simulink model "robot"  (R2018a)
settings: Solver=VariableStepAuto  StartTime=0.0  StopTime=5  RelTol=1e-3
values from neighbouring files (symbols this model uses):
  Ko = 1    [data_robot.m]
  Kv = 1    [data_robot.m]
  L = 0.02    [data_maglev.m]    (also in data_robot.m = 15)
  x0 = 10    [data_robot.m]
  y0 = 30    [data_robot.m]    (also in quadcopter optimisation.m = [0, 0]'; t1.m = 0)
settings Model: Creator=st006736  LastModifiedBy=Anton

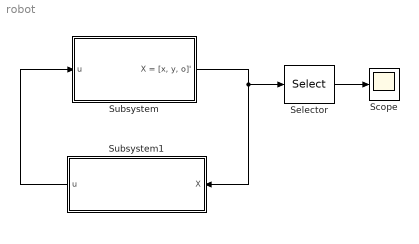
== system robot ==
  Scope : Scope
  Selector : Selector  InputPortWidth=3  IndexOptions=Index vector (dialog)  Indices=[1 2]  OutputSizes=1
  Subsystem : Subsystem
  Subsystem1 : Subsystem
  wires:
  Subsystem/1("X = [x, y, o]'") -> Selector/1, Subsystem1/1(X)
  Subsystem1/1(u) -> Subsystem/1(u)
  Selector/1 -> Scope/1

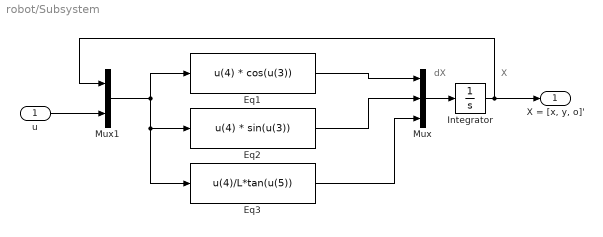
== system robot/Subsystem ==
  note: dX
  note: X
  u : Inport
  Eq1 : Fcn  Expr=u(4) * cos(u(3))
  Eq2 : Fcn  Expr=u(4) * sin(u(3))
  Eq3 : Fcn  Expr=u(4)/L*tan(u(5))
  Integrator : Integrator
  Mux : Mux  Inputs=3
  Mux1 : Mux  Inputs=2
  "X = [x, y, o]'" : Outport
  wires:
  Integrator/1 -> "X = [x, y, o]'"/1, Mux1/1
  Mux/1 -> Integrator/1
  Eq1/1 -> Mux/1
  Eq2/1 -> Mux/2
  Eq3/1 -> Mux/3
  u/1 -> Mux1/2
  Mux1/1 -> Eq1/1, Eq3/1, Eq2/1

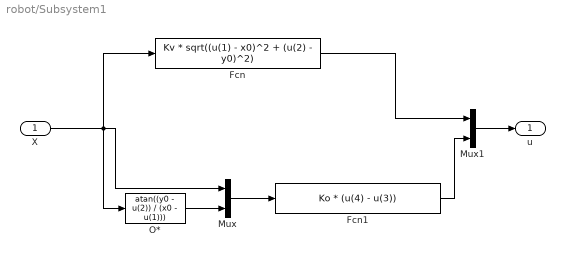
== system robot/Subsystem1 ==
  X : Inport
  Fcn : Fcn  Expr=Kv * sqrt((u(1) - x0)^2 + (u(2) - y0)^2)
  Fcn1 : Fcn  Expr=Ko * (u(4) - u(3))
  Mux : Mux  Inputs=2
  Mux1 : Mux  Inputs=2
  O* : Fcn  Expr=atan((y0 - u(2)) / (x0 - u(1)))
  u : Outport
  wires:
  X/1 -> Mux/1, Fcn/1, O*/1
  O*/1 -> Mux/2
  Mux/1 -> Fcn1/1
  Mux1/1 -> u/1
  Fcn/1 -> Mux1/1
  Fcn1/1 -> Mux1/2
